simulink model "Data Transmission System"  (R2021a)
settings: Solver=VariableStepAuto  StartTime=0.0  StopTime=10.0  MaxStep=0.0001  MinStep=0.0000001  RelTol=1e-3
libraries: commutil2 x8, dspquant2 x8, dsparch4 x4, dspsigops x4, commdigbbndpm3 x2
settings Model: Creator=nisha  LastModifiedBy=nisha

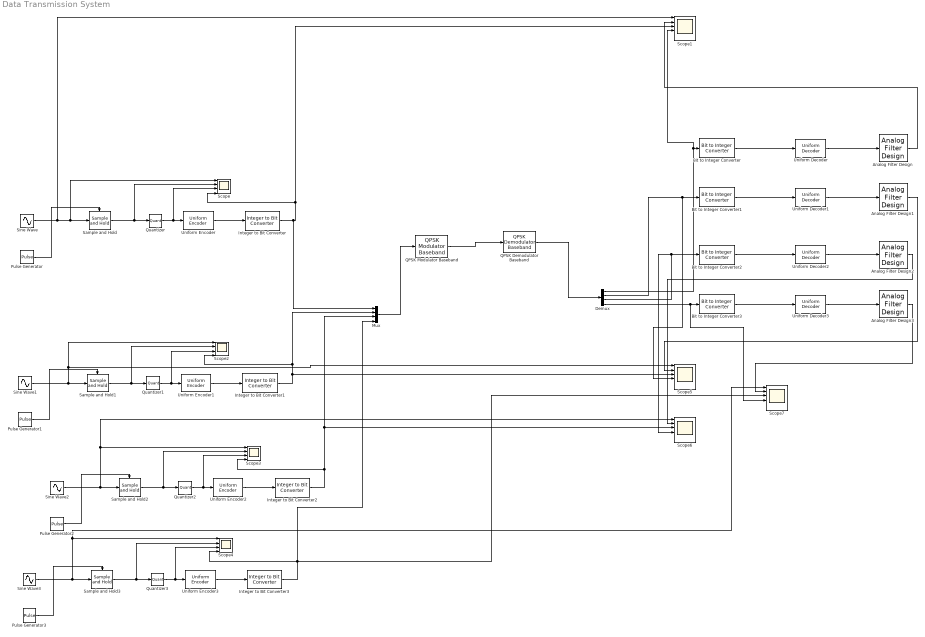
== system Data Transmission System ==
  Analog Filter Design : dsparch4/Analog Filter Design  method=Butterworth  filttype=Lowpass  N=2  Wlo=2*pi*2000  Whi=80  Rp=2  Rs=40
  Analog Filter Design1 : dsparch4/Analog Filter Design  method=Butterworth  filttype=Lowpass  N=2  Wlo=2*pi*5000  Whi=80  Rp=2  Rs=40
  Analog Filter Design2 : dsparch4/Analog Filter Design  method=Butterworth  filttype=Lowpass  N=2  Wlo=2*pi*4000  Whi=80  Rp=2  Rs=40
  Analog Filter Design3 : dsparch4/Analog Filter Design  method=Butterworth  filttype=Lowpass  N=2  Wlo=2*pi*4000  Whi=80  Rp=2  Rs=40
  Bit to Integer Converter{,1..3} (4 alike) : commutil2/Bit to Integer Converter  nbits=4  bitOrder=MSB first  signedOutputValues=Signed  outDtype=Inherit via internal rule  outDtypeSigned=int16
  Demux : Demux
  Integer to Bit Converter{,1..3} (4 alike) : commutil2/Integer to Bit Converter  nbits=4  signedInputValues=Signed  bitOrder=MSB first  outDtype=boolean
  Mux : Mux
  Pulse Generator{,1..3} (4 alike) : DiscretePulseGenerator  PulseType=Time based  Period=1/30000  PulseWidth=50  SampleTime=1/12000
  QPSK Demodulator Baseband : commdigbbndpm3/QPSK Demodulator Baseband  OutType=Bit  DecType=Hard decision  VarSource=Dialog  Variance=1  Dec=Gray  Ph=pi/4  outDtype1=Inherit via internal rule  outDtype2=Inherit via internal rule  derotateFactorWordLen=16  derotateFactorDataTypeStr=Inherit: Same word length as input  derotateFactorLastDataTypeStr=Inherit: Same word length as input
  QPSK Modulator Baseband : commdigbbndpm3/QPSK Modulator Baseband  InType=Bit  Enc=Gray  Ph=pi/4  outDtype=double  outWordLen=16  outUDDataType=sfix(16)  outFracLenMode=Best precision  outFracLen=15  outDataTypeStr=double  outLastDataTypeStr=double
  Quantizer{,1..3} (4 alike) : Quantizer  QuantizationInterval=0.125
  Sample and Hold{,1..3} (4 alike) : dspsigops/Sample and Hold  trig=Either edge  initCond=0  latchinput=off
  Scope{,2..4} (4 alike) : Scope  NumInputPorts=4
  Scope{1,5..7} (4 alike) : Scope  NumInputPorts=6
  Sine Wave : Sin  Frequency=2*pi*2000  Phase=pi/2  SampleTime=0
  Sine Wave1 : Sin  Frequency=2*pi*5000  Phase=pi/2  SampleTime=0
  Sine Wave2 : Sin  Frequency=2*pi*4000  Phase=pi/2  SampleTime=0
  Sine Wave3 : Sin  Frequency=2*pi*4000  Phase=pi/2  SampleTime=0
  Uniform Decoder{,1..3} (4 alike) : dspquant2/Uniform Decoder  peak=1.5  bits=4  overflowMode=Saturate  otype=Double
      settings: SourceProductBaseCode=DS
  Uniform Encoder{,1..3} (4 alike) : dspquant2/Uniform Encoder  peak=1  bits=4  otype=Signed integer
  wires:
  Uniform Encoder/1 -> Integer to Bit Converter/1
  Sample and Hold/1 -> Scope/2, Quantizer/1
  Sine Wave/1 -> Scope1/1, Scope/1, Sample and Hold/1
  Pulse Generator/1 -> Sample and Hold/Trigger
  Integer to Bit Converter/1 -> Mux/1, Scope1/3, Scope/4
  Quantizer/1 -> Scope/3, Uniform Encoder/1
  Uniform Decoder/1 -> Analog Filter Design/1
  Bit to Integer Converter/1 -> Uniform Decoder/1
  Analog Filter Design/1 -> Scope1/2
  QPSK Modulator Baseband/1 -> QPSK Demodulator Baseband/1
  Pulse Generator1/1 -> Sample and Hold1/Trigger
  Sine Wave1/1 -> Scope5/1, Scope2/1, Sample and Hold1/1
  Sample and Hold1/1 -> Scope2/2, Quantizer1/1
  Quantizer1/1 -> Scope2/3, Uniform Encoder1/1
  Uniform Encoder1/1 -> Integer to Bit Converter1/1
  Integer to Bit Converter1/1 -> Scope5/3, Mux/2, Scope2/4
  Pulse Generator2/1 -> Sample and Hold2/Trigger
  Sine Wave2/1 -> Scope6/1, Scope3/1, Sample and Hold2/1
  Sample and Hold2/1 -> Scope3/2, Quantizer2/1
  Quantizer2/1 -> Scope3/3, Uniform Encoder2/1
  Uniform Encoder2/1 -> Integer to Bit Converter2/1
  Integer to Bit Converter2/1 -> Scope6/3, Mux/3, Scope3/4
  Pulse Generator3/1 -> Sample and Hold3/Trigger
  Sine Wave3/1 -> Scope7/1, Scope4/1, Sample and Hold3/1
  Sample and Hold3/1 -> Scope4/2, Quantizer3/1
  Quantizer3/1 -> Scope4/3, Uniform Encoder3/1
  Uniform Encoder3/1 -> Integer to Bit Converter3/1
  Integer to Bit Converter3/1 -> Scope7/3, Mux/4, Scope4/4
  Mux/1 -> QPSK Modulator Baseband/1
  QPSK Demodulator Baseband/1 -> Demux/1
  Demux/1 -> Scope1/4, Bit to Integer Converter/1
  Bit to Integer Converter1/1 -> Uniform Decoder1/1
  Uniform Decoder1/1 -> Analog Filter Design1/1
  Bit to Integer Converter2/1 -> Uniform Decoder2/1
  Uniform Decoder2/1 -> Analog Filter Design2/1
  Bit to Integer Converter3/1 -> Uniform Decoder3/1
  Uniform Decoder3/1 -> Analog Filter Design3/1
  Demux/2 -> Scope5/4, Bit to Integer Converter1/1
  Demux/3 -> Bit to Integer Converter2/1, Scope6/4
  Demux/4 -> Scope7/4, Bit to Integer Converter3/1
  Analog Filter Design1/1 -> Scope5/2
  Analog Filter Design2/1 -> Scope6/2
  Analog Filter Design3/1 -> Scope7/2
